simulink model "Circuit_Diagram"  (R2020b)
settings: Solver=VariableStepAuto  StartTime=0.0  StopTime=0.02  RelTol=1e-6
values from neighbouring files (symbols this model uses):
  clock_frequency = 10e6    (= 10000000)    [inv_sim.m]
  counter_bits = 12    [inv_sim.m]
  Ts = 2e-6    (= 2e-06)    [inv_sim.m]
libraries: ee_lib x18, nesl_utility x17, fl_lib x12, simulink x4
settings Model: Creator=ge62gas  LastModifiedBy=ge62gas

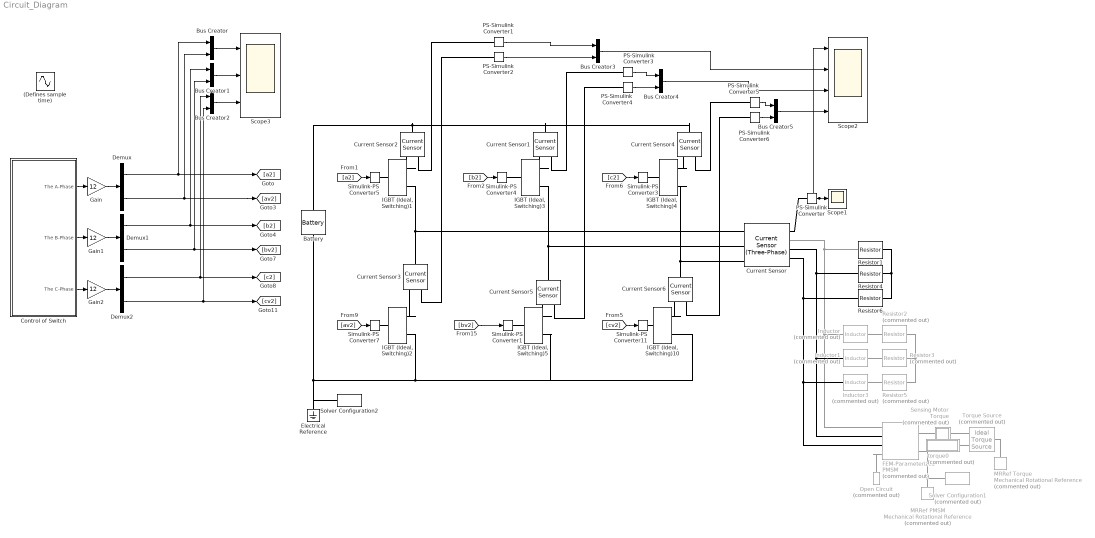
== system Circuit_Diagram ==
  (Defines sample time) : Sin  SampleTime=1e-6
  Battery : ee_lib/Sources/Battery  Vnom=400 V  prm_dir=1  R1_dis=2 Ohm  R1_ch=2 Ohm  R1=2 Ohm  prm_AH=1  AH=50 hr*A  V1=11.5 V  AH1=25 hr*A  prm_R2=1  R2=2000 Ohm  prm_dyn=1  Rp1=0.005 Ohm  tau1=30 s  Rp2=0.005 Ohm  tau2=30 s  Rp3=0.005 Ohm  tau3=30 s  Rp4=0.005 Ohm  tau4=30 s  Rp5=0.005 Ohm  tau5=30 s  prm_fade=1  N_fade=100  AH_fade=45 hr*A  R1_fade=2.02 Ohm  R1_ch_fade=2.02 Ohm  V1_fade=10.35 V  i_specify=off  i_priority=None  i=0 A  i_nominal_specify=off  i_nominal_unit=A  i_nominal_value=1  v_specify=off  v_priority=None  v=0 V  v_nominal_specify=off  v_nominal_unit=V  v_nominal_value=1  charge_specify=off  charge_priority=High  charge=50 hr*A  charge_nominal_specify=off  charge_nominal_unit=hr*A  charge_nominal_value=1  num_cycles_specify=off  num_cycles_priority=High  num_cycles=0  num_cycles_nominal_specify=off  num_cycles_nominal_unit=1  num_cycles_nominal_value=1  thermal_mass=30000 J/K  Tmeas=298.15 K  Vnom_T2=12 V  R1_T2=2.2 Ohm  R1_T2_dis=2.2 Ohm  R1_T2_ch=2.2 Ohm  V1_T2=11.4 V  R2_T2=2200 Ohm  Rp1_T2=0.005 Ohm  tau1_T2=30 s  Rp2_T2=0.005 Ohm  tau2_T2=30 s  Rp3_T2=0.005 Ohm  tau3_T2=30 s  Rp4_T2=0.005 Ohm  tau4_T2=30 s  Rp5_T2=0.005 Ohm  tau5_T2=30 s  Tmeas2=273.15 K  temperature_specify=off  temperature_priority=High  temperature=298.15 K  temperature_nominal_specify=off  temperature_nominal_unit=K  temperature_nominal_value=1
  Bus Creator{,1..5} (6 alike) : BusCreator  Inputs=2
  Control of Switch : Subsystem
  Current Sensor : ee_lib/Sensors & Transducers/Current Sensor (Three-Phase)
      settings: SourceProductName=Electrical  InternalSimscapePortConfiguration="{\"Bottom\":[],\"Left\":[{\"id\":\"a1\",\"label\":\"a1\",\"type\":\"foundation.electrical.electrical\"},{\"id\":\"b1\",\"label\":\"b1\",\"type\":\"foundation.electrical.electrical\"},{\"id\":\"c1\",\"label\":\"c1\",\"type\":\"foundation.electrical.electrical\"}],\"Right\":[{\"id\":\"I_output\",\"label\":\"I\",\"type\":\"output\"},{\"id\":\"a2\",\"label\":\"a2\",\"type\":\"foundation.electrical.electrical\"},{\"id\":\"b2\",\"label\":\"b2\",\"type\":\"foundation.electrical.electrical\"},{\"id\":\"c2\",\"label\":\"c2\",\"type\":\"foundation.electrical.electrical\"}],\"Top\":[]}"
  Current Sensor{1..6} (6 alike) : fl_lib/Electrical/Electrical Sensors/Current Sensor
  Demux : Demux  Outputs=2
  Demux1 : Demux  Outputs=2
  Demux2 : Demux  Outputs=2
  Electrical Reference : fl_lib/Electrical/Electrical Elements/Electrical Reference
  FEM-Parameterized PMSM : ee_lib/Electromechanical/Permanent Magnet/FEM-Parameterized PMSM  Commented=on  parameterization=1  winding_type=ee.enum.statorconnection.wye  iVec=[-2, 0, 2] A  xVec=[0, 20, 40, 60] deg  dfluxdiMatrix=0.0002 * ones(3, 4) Wb/A  dfluxdxMatrix=[0, -.16, .16, 0; 0, -.16, .16, 0; 0, -.16, .16, 0] Wb/rad  calculate_torque_matrix=1  TorqueMatrix=zeros(3, 3, 3, 4) N*m  idVec1=[-200, 0, 200] A  iqVec1=[-200, 0, 200] A  LdMatrix=0.0002 * ones(3, 3) H  LqMatrix=0.0002 * ones(3, 3) H  PmMatrix=0.1 * ones(3, 3) Wb  N=6  interp_method=simscape.enum.interpolation.linear  Rs=0.13 Ohm  Ms=0.0002 H  L0=0.00016 H  losses_oc=[0, 0, 0] W  losses_sc=[0, 0, 0] W  f_losses=60 Hz  Isc_losses=95 A  Inertia=0.1 kg*m^2  lam=0 N*m/(rad/s)  i_d_specify=off  i_d_priority=None  i_d=0 A  i_d_nominal_specify=off  i_d_nominal_unit=A  i_d_nominal_value=1  i_q_specify=off  i_q_priority=None  i_q=0 A  i_q_nominal_specify=off  i_q_nominal_unit=A  i_q_nominal_value=1  torque_specify=off  torque_priority=None  torque=0 N*m  torque_nominal_specify=off  torque_nominal_unit=N*m  torque_nominal_value=1  angular_velocity_specify=off  angular_velocity_priority=High  angular_velocity=0 rpm  angular_velocity_nominal_specify=off  angular_velocity_nominal_unit=rpm  angular_velocity_nominal_value=1  angular_position_specify=off  angular_position_priority=High  angular_position=0 deg  angular_position_nominal_specify=off  angular_position_nominal_unit=deg  angular_position_nominal_value=1  Tmeas=298.15 K  alpha=3.93e-3 1/K  alpha_flux=-0.001 1/K  stator_thermal_mass=100 J/K  stator_initial_temperatures=[298.15, 298.15, 298.15] K  rotor_thermal_mass=200 J/K  rotor_initial_temperature=298.15 K  Rm_percent_rotor=90  Rd_percent_rotor=30  idVec=[-200, 0, 200] A  iqVec=[-200, 0, 200] A  dfluxAdiaMatrix3D=zeros(3, 3, 4) Wb/A  dfluxAdibMatrix3D=zeros(3, 3, 4) Wb/A  dfluxAdicMatrix3D=zeros(3, 3, 4) Wb/A  dfluxAdxMatrix3D=zeros(3, 3, 4) Wb/rad  TorqueMatrix3D=zeros(3, 3, 4) N*m  iaVec=[-200, 0, 200] A  ibVec=[-200, 0, 200] A  icVec=[-200, 0, 200] A  dfluxAdiaMatrix=zeros(3, 3, 3, 4) Wb/A  dfluxAdibMatrix=zeros(3, 3, 3, 4) Wb/A  dfluxAdicMatrix=zeros(3, 3, 3, 4) Wb/A  dfluxAdxMatrix=zeros(3, 3, 3, 4) Wb/rad  param_dq0=1  winding_type_dq0=ee.enum.statorconnection.wye  nPolePairs=4  parks_type=1  idVec2=[-200, 0, 200] A  iqVec2=[-200, 0, 200] A  magVec2=[0, 100, 200] A  betaVec2=[-180, -90, 0, 90, 180] deg  xVec2=[0, 5, 10, 15, 20, 25, 30] deg  fluxD_dq0=zeros(3, 3, 7) Wb  fluxQ_dq0=zeros(3, 3, 7) Wb  fluxA_dq0=zeros(3, 3, 7) Wb  Torque_dq0=zeros(3, 3, 7) N*m  fluxD_IBX=zeros(3, 5, 7) Wb  fluxQ_IBX=zeros(3, 5, 7) Wb  fluxA_IBX=zeros(3, 5, 7) Wb  Torque_IBX=zeros(3, 5, 7) N*m
      settings: SourceProductBaseCode=PS  InternalSimscapePortConfiguration="{\"Bottom\":[],\"Left\":[{\"id\":\"a\",\"label\":\"a\",\"type\":\"foundation.electrical.electrical\"},{\"id\":\"b\",\"label\":\"b\",\"type\":\"foundation.electrical.electrical\"},{\"id\":\"c\",\"label\":\"c\",\"type\":\"foundation.electrical.electrical\"},{\"id\":\"n\",\"label\":\"n\",\"type\":\"foundation.electrical.electrical\"}],\"Right\":[{\"id\":\"R\",\"label\":\"R\",\"type\":\"foundation.mechanical.rotational.rotational\"},{\"id\":\"C\",\"label\":\"C\",\"type\":\"foundation.mechanical.rotational.rotational\"}],\"Top\":[]}"
  Gain : Gain  Gain=12
  Gain1 : Gain  Gain=12
  Gain2 : Gain  Gain=12
  IGBT (Ideal, Switching){1..5,10} (6 alike) : ee_lib/Semiconductors & Converters/IGBT (Ideal, Switching)  Vf=0.8 V  Ron=0.001 Ohm  Goff=1e-5 1/Ohm  Vth=6 V  diode_param=ee.enum.converters.protectiondiode.none  diode_Vf=0.8 V  diode_Ron=0.001 Ohm  diode_Goff=1e-5 1/Ohm  diode_C=50e-9 F  diode_iRM=-235 A  diode_iF=300 A  diode_idot=-50 A/us  diode_trr_param=ee.enum.converters.diodetrr.trr_factor  diode_trr_factor=3  diode_trr=15 us  diode_Qrr=1500 s*uA  thermal_loss_option=ee.enum.converters.thermalLossOption.constantvalues  Von_data=[0, .1, .6, .8, 1, 1.3, 1.6, 2, 2.4; 0, .1, .7, 1, 1.2, 1.5, 1.9, 2.4, 2.8] V  Eon_data=[0, .0024, .024, .12, .2, .48, 1.04, 2.16, 3.24; 0, .003, .03, .15, .25, .6, 1.3, 2.7, 4.05] * 1e-3 J  Eoff_data=[0, .0007, .0066, .033, .066, .17, .33, .83, 1.5; 0, .001, .01, .05, .1, .25, .5, 1.2, 2.2] * 1e-3 J  Tj=[298.15, 398.15] K  Iout_data=[0, .1, 1, 5, 10, 20, 40, 70, 100] A  Eon_scalar=22.86e-3 J  Eoff_scalar=17.14e-3 J  Voff=300 V  Iout_scalar=600 A  diodeModelType=ee.enum.converters.diodeModelType.pwl  diode_IfMat=[.07, .12, .19, 1.75, 4.24, 7.32, 11.2; .16, .3, .72, 2.14, 4.02, 6.35, 9.12] A  diode_TjVec=[25, 125] degC  diode_VfVec=[.5, .7, .9, 1.3, 1.7, 2.1, 2.5] V  thermal_network_parameterization=ee.enum.thermalNetworkTopology.external  Rth=[.08, .5] K/W  Rth_Foster=[.08, .14, .22, .16] K/W  thermal_mass_parameterization=ee.enum.thermalNetwork.timeconstant  thermal_mass=[.01, .5] J/K  thermal_mass_Foster=[.001, .005, .05, .5] J/K  thermal_time_constant=[.001, .2] s  thermal_time_constant_Foster=[7e-05, .0007, .01, .08] s  thermal_mass_initial_temperatures=[25, 25] degC  junction_thermal_mass=0.01 J/K  Tau=1e-4 s  vT_specify=off  vT_priority=None  vT=0 V  vT_nominal_specify=off  vT_nominal_unit=V  vT_nominal_value=1  Qj_specify=off  Qj_priority=None  Qj=0 W  Qj_nominal_specify=off  Qj_nominal_unit=W  Qj_nominal_value=1  junction_temperature_specify=off  junction_temperature_priority=None  junction_temperature=25 degC  junction_temperature_nominal_specify=off  junction_temperature_nominal_unit=degC  junction_temperature_nominal_value=1
  Inductor : ee_lib/Passive/Inductor  Commented=on  l=1e-6 H  L_tol=20  enable_L_tol=0  tol_distribution=1  nSigma=4  r=0 Ohm  g=1e-9 1/Ohm  enable_operating_limits=0  operating_limit_action=2  max_working_current=1 A  power_rating=1 W  enable_faults=0  fault_action=1  lambdaPercent=50  k_faulted=0.9999  turnsShort=0  openCct=0  groundShort=0  groundShortG=0 1/Ohm  tau_fault=1e-3 s  enable_temporal_fault=0  t_fault=1 s  enable_behavioral_fault=0  max_permissible_voltage=100 V  n_fail_on_voltage=1  max_permissible_current=1 A  t_fail_on_current=1 s  i_L_specify=off  i_L_priority=High  i_L=0 A  i_L_nominal_specify=off  i_L_nominal_unit=A  i_L_nominal_value=1
  Inductor1 : ee_lib/Passive/Inductor  Commented=on  l=1e-6 H  L_tol=20  enable_L_tol=0  tol_distribution=1  nSigma=4  r=0 Ohm  g=1e-9 1/Ohm  enable_operating_limits=0  operating_limit_action=2  max_working_current=1 A  power_rating=1 W  enable_faults=0  fault_action=1  lambdaPercent=50  k_faulted=0.9999  turnsShort=0  openCct=0  groundShort=0  groundShortG=0 1/Ohm  tau_fault=1e-3 s  enable_temporal_fault=0  t_fault=1 s  enable_behavioral_fault=0  max_permissible_voltage=100 V  n_fail_on_voltage=1  max_permissible_current=1 A  t_fail_on_current=1 s  i_L_specify=off  i_L_priority=High  i_L=0 A  i_L_nominal_specify=off  i_L_nominal_unit=A  i_L_nominal_value=1
  Inductor3 : ee_lib/Passive/Inductor  Commented=on  l=1e-6 H  L_tol=20  enable_L_tol=0  tol_distribution=1  nSigma=4  r=0 Ohm  g=1e-9 1/Ohm  enable_operating_limits=0  operating_limit_action=2  max_working_current=1 A  power_rating=1 W  enable_faults=0  fault_action=1  lambdaPercent=50  k_faulted=0.9999  turnsShort=0  openCct=0  groundShort=0  groundShortG=0 1/Ohm  tau_fault=1e-3 s  enable_temporal_fault=0  t_fault=1 s  enable_behavioral_fault=0  max_permissible_voltage=100 V  n_fail_on_voltage=1  max_permissible_current=1 A  t_fail_on_current=1 s  i_L_specify=off  i_L_priority=High  i_L=0 A  i_L_nominal_specify=off  i_L_nominal_unit=A  i_L_nominal_value=1
  MRRef PMSM : fl_lib/Mechanical/Rotational Elements/Mechanical Rotational Reference  Commented=on
      settings: SourceProductName=Foundation Library
  MRRef Torque : fl_lib/Mechanical/Rotational Elements/Mechanical Rotational Reference  Commented=on
      settings: SourceProductName=Foundation Library
  Open Circuit : fl_lib/Electrical/Electrical Elements/Open Circuit  Commented=on  v_specify=off  v_priority=None  v=0 V  v_nominal_specify=off  v_nominal_unit=V  v_nominal_value=1
      settings: SourceProductName=Foundation Library
  PS-Simulink Converter{,1..6} (7 alike) : nesl_utility/PS-Simulink Converter  PhysicalDomain=network_engine_domain  SubClassName=ps_output  LeftPortType=input  RightPortType=output  PseudoPeriodic=off  Frequencies=[]  Unit=A  AffineConversion=off
      settings: SourceProductName=Utilities
  Resistor1 : ee_lib/Passive/Resistor  R=0.13 Ohm  R_tol=5  enable_R_tol=0  tol_distribution=1  nSigma=4  enable_operating_limits=0  operating_limit_action=2  max_working_voltage=100 V  power_rating=1 W  enable_faults=0  fault_action=1  R_faulted=inf Ohm  enable_temporal_fault=0  t_fault=1 s  enable_behavioral_fault=0  max_permissible_current=1 A  t_fail_on_current=1 s  noise_mode=0  sample_time=1e-3 s  repeatability=1  auto_seed=2696827909  user_seed=0  Tdevice=25 degC  alpha=3.93e-3 1/K  Tmeas=25 degC  thermal_mass=100 J/K  power_derating_T1=70 degC  power_derating_T2=155 degC  operating_temperature_range_vec=[-50, 150] degC  temperature_specify=off  temperature_priority=High  temperature=298.15 K  temperature_nominal_specify=off  temperature_nominal_unit=K  temperature_nominal_value=1
  Resistor2 : ee_lib/Passive/Resistor  Commented=on  R=0.13 Ohm  R_tol=5  enable_R_tol=0  tol_distribution=1  nSigma=4  enable_operating_limits=0  operating_limit_action=2  max_working_voltage=100 V  power_rating=1 W  enable_faults=0  fault_action=1  R_faulted=inf Ohm  enable_temporal_fault=0  t_fault=1 s  enable_behavioral_fault=0  max_permissible_current=1 A  t_fail_on_current=1 s  noise_mode=0  sample_time=1e-3 s  repeatability=1  auto_seed=3679311552  user_seed=0  Tdevice=25 degC  alpha=3.93e-3 1/K  Tmeas=25 degC  thermal_mass=100 J/K  power_derating_T1=70 degC  power_derating_T2=155 degC  operating_temperature_range_vec=[-50, 150] degC  temperature_specify=off  temperature_priority=High  temperature=298.15 K  temperature_nominal_specify=off  temperature_nominal_unit=K  temperature_nominal_value=1
  Resistor3 : ee_lib/Passive/Resistor  Commented=on  R=0.13 Ohm  R_tol=5  enable_R_tol=0  tol_distribution=1  nSigma=4  enable_operating_limits=0  operating_limit_action=2  max_working_voltage=100 V  power_rating=1 W  enable_faults=0  fault_action=1  R_faulted=inf Ohm  enable_temporal_fault=0  t_fault=1 s  enable_behavioral_fault=0  max_permissible_current=1 A  t_fail_on_current=1 s  noise_mode=0  sample_time=1e-3 s  repeatability=1  auto_seed=1650614420  user_seed=0  Tdevice=25 degC  alpha=3.93e-3 1/K  Tmeas=25 degC  thermal_mass=100 J/K  power_derating_T1=70 degC  power_derating_T2=155 degC  operating_temperature_range_vec=[-50, 150] degC  temperature_specify=off  temperature_priority=High  temperature=298.15 K  temperature_nominal_specify=off  temperature_nominal_unit=K  temperature_nominal_value=1
  Resistor4 : ee_lib/Passive/Resistor  R=0.13 Ohm  R_tol=5  enable_R_tol=0  tol_distribution=1  nSigma=4  enable_operating_limits=0  operating_limit_action=2  max_working_voltage=100 V  power_rating=1 W  enable_faults=0  fault_action=1  R_faulted=inf Ohm  enable_temporal_fault=0  t_fault=1 s  enable_behavioral_fault=0  max_permissible_current=1 A  t_fail_on_current=1 s  noise_mode=0  sample_time=1e-3 s  repeatability=1  auto_seed=1934402393  user_seed=0  Tdevice=25 degC  alpha=3.93e-3 1/K  Tmeas=25 degC  thermal_mass=100 J/K  power_derating_T1=70 degC  power_derating_T2=155 degC  operating_temperature_range_vec=[-50, 150] degC  temperature_specify=off  temperature_priority=High  temperature=298.15 K  temperature_nominal_specify=off  temperature_nominal_unit=K  temperature_nominal_value=1
  Resistor5 : ee_lib/Passive/Resistor  Commented=on  R=0.13 Ohm  R_tol=5  enable_R_tol=0  tol_distribution=1  nSigma=4  enable_operating_limits=0  operating_limit_action=2  max_working_voltage=100 V  power_rating=1 W  enable_faults=0  fault_action=1  R_faulted=inf Ohm  enable_temporal_fault=0  t_fault=1 s  enable_behavioral_fault=0  max_permissible_current=1 A  t_fail_on_current=1 s  noise_mode=0  sample_time=1e-3 s  repeatability=1  auto_seed=2987969779  user_seed=0  Tdevice=25 degC  alpha=3.93e-3 1/K  Tmeas=25 degC  thermal_mass=100 J/K  power_derating_T1=70 degC  power_derating_T2=155 degC  operating_temperature_range_vec=[-50, 150] degC  temperature_specify=off  temperature_priority=High  temperature=298.15 K  temperature_nominal_specify=off  temperature_nominal_unit=K  temperature_nominal_value=1
  Resistor6 : ee_lib/Passive/Resistor  R=0.13 Ohm  R_tol=5  enable_R_tol=0  tol_distribution=1  nSigma=4  enable_operating_limits=0  operating_limit_action=2  max_working_voltage=100 V  power_rating=1 W  enable_faults=0  fault_action=1  R_faulted=inf Ohm  enable_temporal_fault=0  t_fault=1 s  enable_behavioral_fault=0  max_permissible_current=1 A  t_fail_on_current=1 s  noise_mode=0  sample_time=1e-3 s  repeatability=1  auto_seed=2034173572  user_seed=0  Tdevice=25 degC  alpha=3.93e-3 1/K  Tmeas=25 degC  thermal_mass=100 J/K  power_derating_T1=70 degC  power_derating_T2=155 degC  operating_temperature_range_vec=[-50, 150] degC  temperature_specify=off  temperature_priority=High  temperature=298.15 K  temperature_nominal_specify=off  temperature_nominal_unit=K  temperature_nominal_value=1
  Scope1 : Scope
  Scope2 : Scope  NumInputPorts=4
  Scope3 : Scope  NumInputPorts=3
  Sensing Motor Torque : Subsystem  Commented=on
      mask Display: disp('trq');
  Simulink-PS Converter{1,3..5,7,11} (6 alike) : nesl_utility/Simulink-PS Converter  PhysicalDomain=network_engine_domain  SubClassName=ps_input  LeftPortType=input  RightPortType=output  PseudoPeriodic=off  Frequencies=[]  NoiseDistribution=none  NoiseParameters=[]  Unit=1  AffineConversion=off  FilteringAndDerivatives=provide  SimscapeFilterOrder=1  InputFilterTimeConstant=0.001  UdotUserProvided=0
  Solver Configuration1 : nesl_utility/Solver Configuration  Commented=on  PhysicalDomain=network_engine_domain  SubClassName=solver  LeftPortType=input  RightPortType=generic  Tones=[]  Harmonics=[]  SimulateNoise=off  Profile=off  UseLocalSampling=off  EnableSwitchedLinearOptims=on  FrequencyDomain=off  UseCCode=off  RelTol=0.001  AbsTol=1e-06  MinStep=1e-09  ToWorkspace=off  RevertToSquareIcSolve=off  NumHomotopyIterations=100  PhasorMode=off  PhasorModeNumHarmonics=1  DoDC=off  ResidualTolerance=1e-9  UseLocalSolver=off  LocalSolverChoice=NE_BACKWARD_EULER_ADVANCER  LocalSolverSampleTime=Ts/1000  DoFixedCost=on  MaxNonlinIter=4  MaxModeIter=2  ComputeImpulses=off  ImpulseIterations=2  LinearAlgebra=auto  EquationFormulation=NE_TIME_EF  DelaysMemoryBudget=1024  AutomaticFiltering=on  FilteringTimeConstant=0.001  PartitionStorageMethod=AS_NEEDED  PartitionMemoryBudget=1024  PartitionMethod=FAST
      settings: SourceProductName=Utilities
  Solver Configuration2 : nesl_utility/Solver Configuration  PhysicalDomain=network_engine_domain  SubClassName=solver  LeftPortType=input  RightPortType=generic  Tones=[]  Harmonics=[]  SimulateNoise=off  Profile=off  UseLocalSampling=off  EnableSwitchedLinearOptims=on  FrequencyDomain=off  UseCCode=off  RelTol=0.001  AbsTol=1e-06  MinStep=1e-09  ToWorkspace=off  RevertToSquareIcSolve=off  NumHomotopyIterations=100  PhasorMode=off  PhasorModeNumHarmonics=1  DoDC=off  ResidualTolerance=1e-9  UseLocalSolver=off  LocalSolverChoice=NE_BACKWARD_EULER_ADVANCER  LocalSolverSampleTime=Ts/1000  DoFixedCost=on  MaxNonlinIter=4  MaxModeIter=2  ComputeImpulses=off  ImpulseIterations=2  LinearAlgebra=auto  EquationFormulation=NE_TIME_EF  DelaysMemoryBudget=1024  AutomaticFiltering=on  FilteringTimeConstant=0.001  PartitionStorageMethod=AS_NEEDED  PartitionMemoryBudget=1024  PartitionMethod=FAST
      settings: SourceProductName=Utilities
  Torque Source : fl_lib/Mechanical/Mechanical Sources/Ideal Torque Source  Commented=on
      settings: SourceProductName=Foundation Library
  torque0 : Subsystem  Commented=on
      mask Display: disp('torque0');
  wires:
  Demux/1 -> Bus Creator/1, [a2]
  Demux/2 -> [av2], Bus Creator/2
  Demux1/1 -> Bus Creator1/1, [b2]
  Demux1/2 -> Bus Creator1/2, [bv2]
  Demux2/1 -> Bus Creator2/1, [c2]
  Demux2/2 -> [cv2], Bus Creator2/2
  [c2] -> Simulink-PS Converter3/1
  [cv2] -> Simulink-PS Converter11/1
  [a2] -> Simulink-PS Converter5/1
  PS-Simulink Converter/1 -> Scope2/1, Scope1/1
  [av2] -> Simulink-PS Converter7/1
  [b2] -> Simulink-PS Converter4/1
  PS-Simulink Converter2/1 -> Bus Creator3/2
  PS-Simulink Converter1/1 -> Bus Creator3/1
  Gain1/1 -> Demux1/1
  Control of Switch/3(The C-Phase) -> Gain2/1
  Control of Switch/2(The B-Phase) -> Gain1/1
  Gain2/1 -> Demux2/1
  Control of Switch/1(The A-Phase) -> Gain/1
  Gain/1 -> Demux/1
  Bus Creator/1 -> Scope3/1
  Bus Creator1/1 -> Scope3/2
  Bus Creator2/1 -> Scope3/3
  Bus Creator3/1 -> Scope2/2
  PS-Simulink Converter3/1 -> Bus Creator4/1
  PS-Simulink Converter4/1 -> Bus Creator4/2
  Bus Creator4/1 -> Scope2/3
  PS-Simulink Converter6/1 -> Bus Creator5/2
  PS-Simulink Converter5/1 -> Bus Creator5/1
  Bus Creator5/1 -> Scope2/4
  [bv2] -> Simulink-PS Converter1/1
  connections:
  Solver Configuration1/RConn1 -- FEM-Parameterized PMSM/RConn2 -- MRRef PMSM/LConn1
  Current Sensor2/LConn1 -- Current Sensor1/LConn1 -- Current Sensor4/LConn1 -- Battery/LConn1
  "IGBT (Ideal, Switching)2"/RConn2 -- "IGBT (Ideal, Switching)10"/RConn2 -- "IGBT (Ideal, Switching)5"/RConn2 -- Electrical Reference/LConn1 -- Solver Configuration2/RConn1 -- Battery/RConn1
  "IGBT (Ideal, Switching)3"/RConn2 -- Current Sensor/LConn2 -- Current Sensor5/LConn1
  Current Sensor3/LConn1 -- "IGBT (Ideal, Switching)1"/RConn2 -- Current Sensor/LConn1
  "IGBT (Ideal, Switching)4"/RConn2 -- Current Sensor6/LConn1 -- Current Sensor/LConn3
  "IGBT (Ideal, Switching)1"/RConn1 -- Current Sensor2/RConn2
  "IGBT (Ideal, Switching)4"/LConn1 -- Simulink-PS Converter3/RConn1
  Sensing Motor Torque/RConn1 -- Torque Source/RConn2
  torque0/RConn1 -- Torque Source/RConn1
  FEM-Parameterized PMSM/LConn4 -- Open Circuit/LConn1
  FEM-Parameterized PMSM/RConn1 -- Sensing Motor Torque/LConn1
  PS-Simulink Converter/LConn1 -- Current Sensor/RConn1
  Simulink-PS Converter7/RConn1 -- "IGBT (Ideal, Switching)2"/LConn1
  Simulink-PS Converter11/RConn1 -- "IGBT (Ideal, Switching)10"/LConn1
  Simulink-PS Converter5/RConn1 -- "IGBT (Ideal, Switching)1"/LConn1
  MRRef Torque/LConn1 -- Torque Source/LConn1
  "IGBT (Ideal, Switching)2"/RConn1 -- Current Sensor3/RConn2
  "IGBT (Ideal, Switching)3"/LConn1 -- Simulink-PS Converter4/RConn1
  PS-Simulink Converter1/LConn1 -- Current Sensor2/RConn1
  PS-Simulink Converter2/LConn1 -- Current Sensor3/RConn1
  Resistor2/RConn1 -- Resistor3/RConn1 -- Resistor5/RConn1
  Inductor3/RConn1 -- Resistor5/LConn1
  Inductor1/RConn1 -- Resistor3/LConn1
  Inductor/RConn1 -- Resistor2/LConn1
  Inductor/LConn1 -- Resistor1/LConn1 -- Current Sensor/RConn2 -- FEM-Parameterized PMSM/LConn1
  Current Sensor/RConn3 -- Resistor4/LConn1 -- FEM-Parameterized PMSM/LConn2 -- Inductor1/LConn1
  Current Sensor/RConn4 -- Resistor6/LConn1 -- FEM-Parameterized PMSM/LConn3 -- Inductor3/LConn1
  "IGBT (Ideal, Switching)3"/RConn1 -- Current Sensor1/RConn2
  "IGBT (Ideal, Switching)4"/RConn1 -- Current Sensor4/RConn2
  Current Sensor1/RConn1 -- PS-Simulink Converter3/LConn1
  Current Sensor4/RConn1 -- PS-Simulink Converter5/LConn1
  "IGBT (Ideal, Switching)10"/RConn1 -- Current Sensor6/RConn2
  Current Sensor6/RConn1 -- PS-Simulink Converter6/LConn1
  Resistor4/RConn1 -- Resistor1/RConn1 -- Resistor6/RConn1
  "IGBT (Ideal, Switching)5"/LConn1 -- Simulink-PS Converter1/RConn1
  "IGBT (Ideal, Switching)5"/RConn1 -- Current Sensor5/RConn2
  Current Sensor5/RConn1 -- PS-Simulink Converter4/LConn1

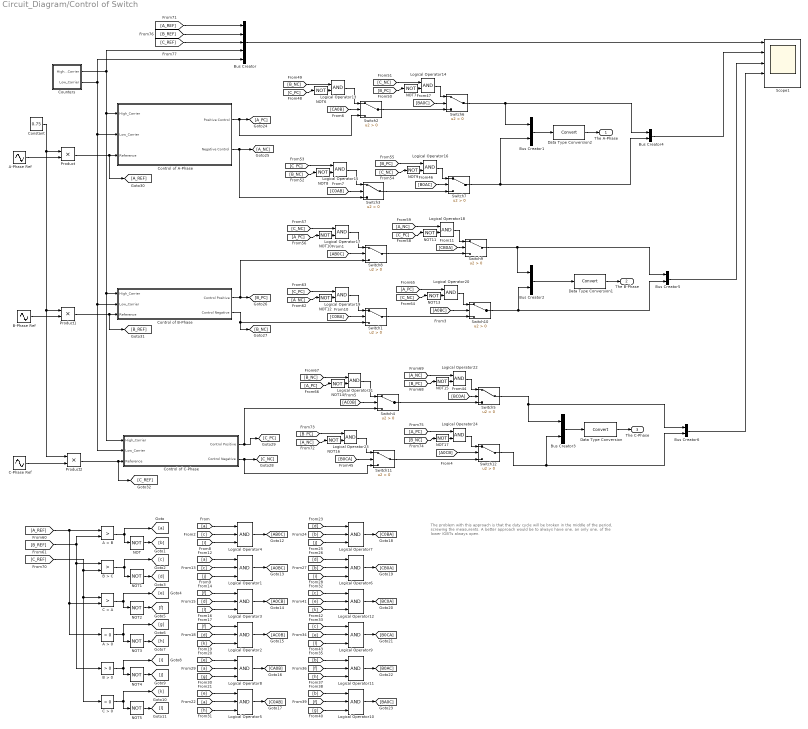
== system Circuit_Diagram/Control of Switch ==
  note: The problem with this approach is that the duty cycle will be broken in the middle of the period, screwing the measurents. A better approach would be to always have one, an only one, of the lower IGBTs always open.
  A > 0 : simulink/Logic and Bit Operations/Compare To Zero  relop=>  OutDataTypeStr=boolean
  A > B : RelationalOperator  Operator=>  OutDataTypeStr=boolean  RndMeth=Simplest
  A-Phase Ref : Sin  Amplitude=2^(counter_bits-1)  Frequency=2*pi*50  SampleTime=0
  B > 0 : simulink/Logic and Bit Operations/Compare To Zero  relop=>  OutDataTypeStr=boolean
  B > C : RelationalOperator  Operator=>  OutDataTypeStr=boolean  RndMeth=Simplest
  B-Phase Ref : Sin  Amplitude=2^(counter_bits-1)  Frequency=2*pi*50  Phase=2*pi/3  SampleTime=0
  Bus Creator : BusCreator  Inputs=5
  Bus Creator{1..6} (6 alike) : BusCreator  Inputs=2
  C > 0 : simulink/Logic and Bit Operations/Compare To Zero  relop=>  OutDataTypeStr=boolean
  C > A : RelationalOperator  Operator=>  OutDataTypeStr=boolean  RndMeth=Simplest
  C-Phase Ref : Sin  Amplitude=2^(counter_bits-1)  Frequency=2*pi*50  Phase=-2*pi/3  SampleTime=0
  Constant : Constant  Value=0.75
  Control of A-Phase : Subsystem
  Control of B-Phase : Subsystem
  Control of C-Phase : Subsystem
  Counters : Subsystem
  Data Type Conversion : DataTypeConversion
  Data Type Conversion1 : DataTypeConversion
  Data Type Conversion2 : DataTypeConversion
  Logical Operator{1..12} (12 alike) : Logic  Inputs=3  AllPortsSameDT=off  OutDataTypeStr=boolean
  Logical Operator{13..24} (12 alike) : Logic  AllPortsSameDT=off  OutDataTypeStr=boolean
  NOT{,1..17} (18 alike) : Logic  Operator=NOT  IconShape=distinctive  AllPortsSameDT=off  OutDataTypeStr=boolean
  Product : Product
  Product1 : Product
  Product2 : Product
  Scope1 : Scope  NumInputPorts=5
  Switch{1..12} (12 alike) : Switch  Criteria=u2 > Threshold
  The A-Phase : Outport
  The B-Phase : Outport  Port=2
  The C-Phase : Outport  Port=3
  wires:
  Bus Creator/1 -> Scope1/1
  Bus Creator3/1 -> Data Type Conversion/1
  Data Type Conversion/1 -> The C-Phase/1
  Bus Creator1/1 -> Data Type Conversion2/1
  Data Type Conversion2/1 -> The A-Phase/1
  Bus Creator2/1 -> Data Type Conversion1/1
  Data Type Conversion1/1 -> The B-Phase/1
  Counters/2(Low_Carrier) -> Bus Creator/5, Control of C-Phase/2(Low_Carrier), Control of B-Phase/2(Low_Carrier), Control of A-Phase/2(Low_Carrier)
  Counters/1(High_Carrier) -> Bus Creator/4, Control of C-Phase/1(High_Carrier), Control of B-Phase/1(High_Carrier), Control of A-Phase/1(High_Carrier)
  Bus Creator4/1 -> Scope1/2
  Bus Creator5/1 -> Scope1/3
  Bus Creator6/1 -> Scope1/4
  A > B/1 -> [a], NOT/1
  NOT/1 -> [b]
  NOT1/1 -> [d]
  B > C/1 -> NOT1/1, [c]
  A > 0/1 -> NOT3/1, [g]
  NOT3/1 -> [h]
  NOT2/1 -> [f]
  C > A/1 -> NOT2/1, [e]
  B > 0/1 -> [i], NOT4/1
  NOT4/1 -> [j]
  NOT5/1 -> [l]
  C > 0/1 -> [k], NOT5/1
  [a] -> Logical Operator4/1
  [c] -> Logical Operator4/2
  [i] -> Logical Operator4/3
  [j] -> Logical Operator1/3
  [c] -> Logical Operator1/2
  [a] -> Logical Operator1/1
  [f] -> Logical Operator2/1
  [d] -> Logical Operator2/2
  [k] -> Logical Operator2/3
  [l] -> Logical Operator3/3
  [d] -> Logical Operator3/2
  [f] -> Logical Operator3/1
  [d] -> Logical Operator7/1
  [b] -> Logical Operator7/2
  [j] -> Logical Operator7/3
  [i] -> Logical Operator6/3
  [b] -> Logical Operator6/2
  [d] -> Logical Operator6/1
  [e] -> Logical Operator5/1
  [a] -> Logical Operator5/2
  [h] -> Logical Operator5/3
  [g] -> Logical Operator8/3
  [a] -> Logical Operator8/2
  [e] -> Logical Operator8/1
  [c] -> Logical Operator12/1
  [e] -> Logical Operator12/2
  [k] -> Logical Operator12/3
  [l] -> Logical Operator9/3
  [e] -> Logical Operator9/2
  [c] -> Logical Operator9/1
  [b] -> Logical Operator10/1
  [f] -> Logical Operator10/2
  [g] -> Logical Operator10/3
  [h] -> Logical Operator11/3
  [f] -> Logical Operator11/2
  [b] -> Logical Operator11/1
  Logical Operator4/1 -> [AB0C]
  Logical Operator1/1 -> [A0BC]
  Logical Operator3/1 -> [A0CB]
  Logical Operator2/1 -> [AC0B]
  Logical Operator6/1 -> [CB0A]
  Logical Operator7/1 -> [C0BA]
  Logical Operator5/1 -> [C0AB]
  Logical Operator8/1 -> [CA0B]
  Logical Operator12/1 -> [BC0A]
  Logical Operator9/1 -> [B0CA]
  Logical Operator11/1 -> [B0AC]
  Logical Operator10/1 -> [BA0C]
  Control of B-Phase/1(Control Positive) -> [B_PC], Switch8/3
  Control of B-Phase/2(Control Negative) -> Switch1/3, [B_NC]
  Control of A-Phase/2(Negative Control) -> Switch3/3, [A_NC]
  Control of A-Phase/1(Positive Control) -> Switch2/3, [A_PC]
  Control of C-Phase/1(Control Positive) -> Switch4/3, [C_PC]
  Control of C-Phase/2(Control Negative) -> Switch11/3, [C_NC]
  [CA0B] -> Switch2/2
  [C0AB] -> Switch3/2
  [BA0C] -> Switch6/2
  Switch2/1 -> Switch6/3
  Switch3/1 -> Switch7/3
  [B0AC] -> Switch7/2
  [B_NC] -> Logical Operator13/1
  NOT6/1 -> Logical Operator13/2
  [C_PC] -> NOT6/1
  Logical Operator13/1 -> Switch2/1
  [B_PC] -> NOT7/1
  NOT7/1 -> Logical Operator14/2
  [C_NC] -> Logical Operator14/1
  Logical Operator14/1 -> Switch6/1
  Switch6/1 -> Bus Creator4/1, Bus Creator1/1
  Logical Operator15/1 -> Switch3/1
  [B_NC] -> NOT8/1
  NOT8/1 -> Logical Operator15/2
  [C_PC] -> Logical Operator15/1
  Logical Operator16/1 -> Switch7/1
  [B_PC] -> Logical Operator16/1
  NOT9/1 -> Logical Operator16/2
  [C_NC] -> NOT9/1
  Switch7/1 -> Bus Creator4/2, Bus Creator1/2
  [C_PC] -> NOT11/1
  NOT11/1 -> Logical Operator18/2
  [A_NC] -> Logical Operator18/1
  Logical Operator18/1 -> Switch9/1
  [C_NC] -> Logical Operator17/1
  NOT10/1 -> Logical Operator17/2
  [A_PC] -> NOT10/1
  Logical Operator17/1 -> Switch8/1
  [CB0A] -> Switch9/2
  Switch8/1 -> Switch9/3
  [AB0C] -> Switch8/2
  Switch9/1 -> Bus Creator2/1, Bus Creator5/1
  [C0BA] -> Switch1/2
  Switch1/1 -> Switch10/3
  [A0BC] -> Switch10/2
  Logical Operator19/1 -> Switch1/1
  [A_NC] -> NOT12/1
  NOT12/1 -> Logical Operator19/2
  [C_PC] -> Logical Operator19/1
  Logical Operator20/1 -> Switch10/1
  [A_PC] -> Logical Operator20/1
  NOT13/1 -> Logical Operator20/2
  [C_NC] -> NOT13/1
  Switch10/1 -> Bus Creator2/2, Bus Creator5/2
  [AC0B] -> Switch4/2
  Switch4/1 -> Switch5/3
  [BC0A] -> Switch5/2
  Logical Operator21/1 -> Switch4/1
  [A_PC] -> NOT14/1
  NOT14/1 -> Logical Operator21/2
  [B_NC] -> Logical Operator21/1
  Logical Operator22/1 -> Switch5/1
  [A_NC] -> Logical Operator22/1
  NOT15/1 -> Logical Operator22/2
  [B_PC] -> NOT15/1
  [B_NC] -> NOT17/1
  NOT17/1 -> Logical Operator24/2
  [A_PC] -> Logical Operator24/1
  Logical Operator24/1 -> Switch12/1
  [B_PC] -> Logical Operator23/1
  NOT16/1 -> Logical Operator23/2
  [A_NC] -> NOT16/1
  Logical Operator23/1 -> Switch11/1
  [A0CB] -> Switch12/2
  Switch11/1 -> Switch12/3
  [B0CA] -> Switch11/2
  Switch5/1 -> Bus Creator3/1, Bus Creator6/1
  Switch12/1 -> Bus Creator6/2, Bus Creator3/2
  [A_REF] -> A > 0/1, C > A/2, A > B/1
  [B_REF] -> B > 0/1, B > C/1, A > B/2
  [C_REF] -> C > 0/1, C > A/1, B > C/2
  [C_REF] -> Bus Creator/3
  [B_REF] -> Bus Creator/2
  [A_REF] -> Bus Creator/1
  Product/1 -> [A_REF], Control of A-Phase/3(Reference)
  A-Phase Ref/1 -> Product/2
  Constant/1 -> Product2/1, Product1/1, Product/1
  B-Phase Ref/1 -> Product1/2
  Product1/1 -> [B_REF], Control of B-Phase/3(Reference)
  Product2/1 -> [C_REF], Control of C-Phase/3(Reference)
  C-Phase Ref/1 -> Product2/2

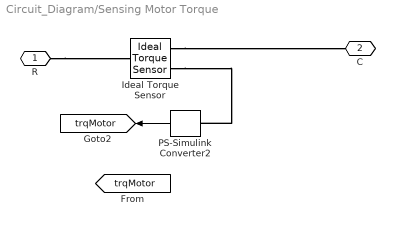
== system Circuit_Diagram/Sensing Motor Torque ==
  Ideal Torque Sensor : fl_lib/Mechanical/Mechanical Sensors/Ideal Torque Sensor
      settings: SourceProductName=Foundation Library
  PS-Simulink Converter2 : nesl_utility/PS-Simulink Converter  PhysicalDomain=network_engine_domain  SubClassName=ps_output  LeftPortType=input  RightPortType=output  PseudoPeriodic=off  Frequencies=[]  Unit=N*m  AffineConversion=off
      settings: SourceProductName=Utilities
  R : PMIOPort  Side=Left
  C : PMIOPort  Port=2  Side=Right
  tag scope: trqMotor=global
  wires:
  PS-Simulink Converter2/1 -> [trqMotor]
  connections:
  Ideal Torque Sensor/RConn2 -- PS-Simulink Converter2/LConn1
  R/RConn1 -- Ideal Torque Sensor/LConn1
  Ideal Torque Sensor/RConn1 -- C/RConn1

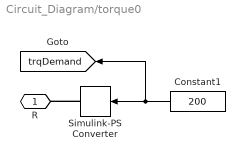
== system Circuit_Diagram/torque0 ==
  Constant1 : Constant  Value=200
  Simulink-PS Converter : nesl_utility/Simulink-PS Converter  PhysicalDomain=network_engine_domain  SubClassName=ps_input  LeftPortType=input  RightPortType=output  PseudoPeriodic=off  Frequencies=[]  NoiseDistribution=none  NoiseParameters=[]  Unit=N*m  AffineConversion=off  FilteringAndDerivatives=zero  SimscapeFilterOrder=1  InputFilterTimeConstant=0.001  UdotUserProvided=1
      settings: SourceProductName=Utilities
  R : PMIOPort  Side=Right
  tag scope: trqDemand=global
  wires:
  Constant1/1 -> Simulink-PS Converter/1, [trqDemand]
  connections:
  Simulink-PS Converter/RConn1 -- R/RConn1

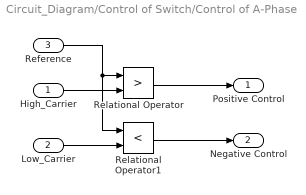
== system Circuit_Diagram/Control of Switch/Control of A-Phase ==
  High_Carrier : Inport
  Low_Carrier : Inport  Port=2
  Reference : Inport  Port=3
  Relational Operator : RelationalOperator  Operator=>  OutDataTypeStr=boolean  RndMeth=Simplest
  Relational Operator1 : RelationalOperator  Operator=<  OutDataTypeStr=boolean  RndMeth=Simplest
  Positive Control : Outport
  Negative Control : Outport  Port=2
  wires:
  Relational Operator/1 -> Positive Control/1
  High_Carrier/1 -> Relational Operator/2
  Reference/1 -> Relational Operator1/1, Relational Operator/1
  Relational Operator1/1 -> Negative Control/1
  Low_Carrier/1 -> Relational Operator1/2

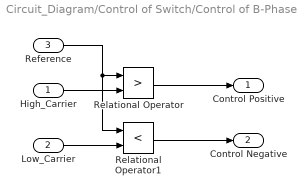
== system Circuit_Diagram/Control of Switch/Control of B-Phase ==
  High_Carrier : Inport
  Low_Carrier : Inport  Port=2
  Reference : Inport  Port=3
  Relational Operator : RelationalOperator  Operator=>  OutDataTypeStr=boolean  RndMeth=Simplest
  Relational Operator1 : RelationalOperator  Operator=<  OutDataTypeStr=boolean  RndMeth=Simplest
  Control Positive : Outport
  Control Negative : Outport  Port=2
  wires:
  Reference/1 -> Relational Operator1/1, Relational Operator/1
  Low_Carrier/1 -> Relational Operator1/2
  High_Carrier/1 -> Relational Operator/2
  Relational Operator/1 -> Control Positive/1
  Relational Operator1/1 -> Control Negative/1

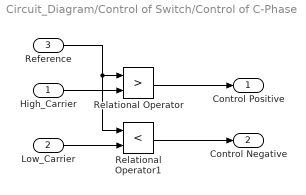
== system Circuit_Diagram/Control of Switch/Control of C-Phase ==
  High_Carrier : Inport
  Low_Carrier : Inport  Port=2
  Reference : Inport  Port=3
  Relational Operator : RelationalOperator  Operator=>  OutDataTypeStr=boolean  RndMeth=Simplest
  Relational Operator1 : RelationalOperator  Operator=<  OutDataTypeStr=boolean  RndMeth=Simplest
  Control Positive : Outport
  Control Negative : Outport  Port=2
  wires:
  Reference/1 -> Relational Operator1/1, Relational Operator/1
  Low_Carrier/1 -> Relational Operator1/2
  High_Carrier/1 -> Relational Operator/2
  Relational Operator/1 -> Control Positive/1
  Relational Operator1/1 -> Control Negative/1

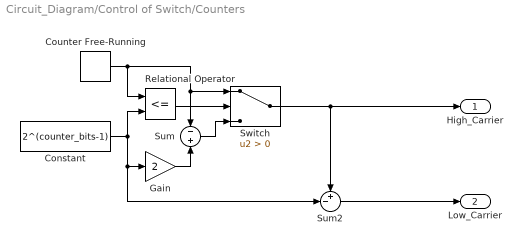
== system Circuit_Diagram/Control of Switch/Counters ==
  Constant : Constant  Value=2^(counter_bits-1)
  Counter Free-Running : simulink/Sources/Counter Free-Running  NumBits=counter_bits  tsamp=1/clock_frequency
  Gain : Gain  Gain=2
  Relational Operator : RelationalOperator  Operator=<=  OutDataTypeStr=boolean  RndMeth=Simplest
  Sum : Sum  Inputs=-|+
  Sum2 : Sum  Inputs=+-|
  Switch : Switch  Criteria=u2 > Threshold
  High_Carrier : Outport
  Low_Carrier : Outport  Port=2
  wires:
  Constant/1 -> Sum2/2, Gain/1, Relational Operator/2
  Relational Operator/1 -> Switch/2
  Sum2/1 -> Low_Carrier/1
  Switch/1 -> High_Carrier/1, Sum2/1
  Sum/1 -> Switch/3
  Gain/1 -> Sum/2
  Counter Free-Running/1 -> Switch/1, Sum/1, Relational Operator/1
